simulink model "LATC_Test_Calc"  (R2021b)
settings: Solver=FixedStepDiscrete  StartTime=0.0  StopTime=inf  FixedStep=0.01  RelTol=1e-3
undefined symbols (not defined in the file or in its folder): P_LCS_A0_Dis_BP, P_LCS_A2_Curve_BP, P_LCS_A2S_FliterTime, P_LCS_DeltaEps_SpdBp, P_LCS_LCC_A0_Dis_BP, P_LCS_LCC_AngleSlope_ELK, P_LCS_LCC_AngleSlope_ESS, P_LCS_LCC_AngleSlope_LCCancle, P_LCS_LCC_AngleSlope_LCEco, P_LCS_LCC_AngleSlope_LCK, P_LCS_LCC_AngleSlope_LCKIE, P_LCS_LCC_AngleSlope_LCNomal, P_LCS_LCC_AngleSlope_LCSport, P_LCS_LCC_AngleSlope_LKA, P_LCS_LCC_Eco_AyDtLimit_TBL, P_LCS_LCC_ELK_AyDtLimit_TBL, P_LCS_LCC_ESS_AyDtLimit_TBL, P_LCS_LCC_LC_AyDtLimit_TBL, P_LCS_LCC_LC_Normal_AyDtLimit_TBL, P_LCS_LCC_LC_Planning_Dist_TBL, P_LCS_LCC_LCK_AyDtLimit_TBL, P_LCS_LCC_LCK_Planning_Dist_TBL, P_LCS_LCC_LKA_AyDtLimit_TBL, P_LCS_LCC_Matrix_q1_st, P_LCS_LCC_Matrix_q2_st, P_LCS_LCC_Max_Lateral_Acc_ms2, P_LCS_LCC_MaxLatAcc_ELK, P_LCS_LCC_MaxLatAcc_ESS, P_LCS_LCC_MaxLatAcc_LCCancel, P_LCS_LCC_MaxLatAcc_LCEco, P_LCS_LCC_MaxLatAcc_LCK, P_LCS_LCC_MaxLatAcc_LCKIE, P_LCS_LCC_MaxLatAcc_LCNomal, P_LCS_LCC_MaxLatAcc_LCSport, P_LCS_LCC_MaxLatAcc_LKA, P_LCS_LCC_Min_Plan_Dis, P_LCS_LCC_PlaningLength_m, P_LCS_LCC_PreCur_Min_Plan_Dis_Fac, P_LCS_LCC_PreView_Fac, P_LCS_LCC_PreView_s, P_LCS_LCC_PreViewCurve_Fac, P_LCS_LCC_PreViewT, P_LCS_LCC_Spd_BP, P_LCS_LCC_Spd_BP2, P_LCS_LCC_Sport_AyDtLimit_TBL, P_LCS_LCC_StateActiv_AyDtLimit, P_LCS_LCC_StateActiv_PreviewT, P_LCS_LCC_StateActiveDelaytime, P_LCS_LCC_TarSteerAngleSlope, P_LCS_preDis_spd, P_LCS_StateActiv_AngleSlope, P_LCS_StateActive_HoldTime_BP, P_LCS_StateActiveFlg_BP, P_LCS_StateHold_time
libraries: canapelib x35, simulink x2
(part 3 of 3)

== matlab function LATC_Test_Calc/MATLAB Function1 ==
  data: LineValid input; SteerAngle input; steer_angle output size=[1,1]; Veh_Speed input; ref_curvature input; lateral_error input; lateral_error_rate input; heading_error input; heading_error_rate input; steer_feedforward_temp output; steer_feedbackward_temp output; Left_steer_ratio input; Right_steer_ratio input; Matrix_q1 input; Matrix_q3 input; Max_lateral_acceleration input; TarSteerAngleSlope input; CurrentSteerAngleOffset input; steer_limit_temp output; steer_angleK1 input
function [steer_angle,steer_feedforward_temp,steer_feedbackward_temp,steer_limit_temp]= LQR_Algorithm(LineValid,SteerAngle,Veh_Speed,ref_curvature,lateral_error,lateral_error_rate,heading_error,heading_error_rate,...
    Left_steer_ratio,Right_steer_ratio,Matrix_q1,Matrix_q3,Max_lateral_acceleration,TarSteerAngleSlope,CurrentSteerAngleOffset,steer_angleK1)
if LineValid
    %% 1.车辆参数
    %1.1 车的大小及长度参数
    veh_params.vehicle_length = single(4.875);
    veh_params.vehicle_width  = single(2.2);
    veh_params.vehicle_height = single(1.69);
    %1.2 车辆控制参数
    veh_params.wheel_base = single(2.92);               %轴距, m
    veh_params.Vch = 23.5;                              %特征车速
    veh_params.max_steer_angle = single(53 / 180 * pi); %前轮最大转角
    veh_params.max_acceleration = single(2);            %车辆最大加速度
    veh_params.max_deceleration = single(-2);           %车辆最大减速度
    veh_params.left_steer_ratio = Left_steer_ratio;     %车辆左侧转向传动比%
    veh_params.right_steer_ratio = Right_steer_ratio;   %车辆右侧转向传动比%
    veh_params.cf = single(155494.663);                 %车辆前轮侧偏刚度
    veh_params.cr = single(155494.663);                 %车辆后轮侧偏刚度 
    veh_params.mass_fl = single(520);                   %车辆左前轮负重
    veh_params.mass_fr = single(520);                   %车辆右前轮负重
    veh_params.mass_rl = single(520);                   %车辆左后轮负重
    veh_params.mass_rr = single(520);                   %车辆右后轮负重
    %% 2.控制参数计算
    mass_front =  veh_params.mass_fl + veh_params.mass_fr;
    mass_rear  =  veh_params.mass_rl + veh_params.mass_rr;
    mass =  mass_front + mass_rear;
    lf = veh_params.wheel_base * (single(1.0) - mass_front / mass);
    lr = veh_params.wheel_base * (single(1.0) - mass_rear / mass);
    iz = lf * lf * mass_front + lr * lr * mass_rear;
    %% 3.LQR参数设置
    
    lqr_eps = single(0.01);
    lqr_max_iteration = single(800);
    
    basic_state_size = uint8(4);
    control_size = uint8(1);
    
    matrix_a=  single(zeros(basic_state_size,basic_state_size));
    matrix_a_coeff = single(zeros(basic_state_size,basic_state_size));
    I = single(eye(basic_state_size,basic_state_size));
    matrix_a(1,2) = single(1.0);
    matrix_a(2,3) = single((veh_params.cf + veh_params.cr ) / mass);
    matrix_a(3,4) = single(1.0);
    matrix_a(4,3) = single((lf * veh_params.cf - lr * veh_params.cr) / iz);
    
    matrix_a_coeff(2,2) = single(-(veh_params.cf + veh_params.cr) / mass);
    matrix_a_coeff(2,4) = single(-1.0 * (lr * veh_params.cr + lf * veh_params.cf) / mass);
    matrix_a_coeff(3,4) = single(1.0);
    matrix_a_coeff(4,2) = single((lr * veh_params.cr - lf * veh_params.cf) / iz);
    matrix_a_coeff(4,4) = single(-1.0 * (lf * lf * veh_params.cf + lr * lr * veh_params.cr)/iz);
    
    matrix_a(2,2) = matrix_a_coeff(2,2);
    matrix_a(2,4) = matrix_a_coeff(2,4);
    matrix_a(4,2) = matrix_a_coeff(4,2);
    matrix_a(4,4) = matrix_a_coeff(4,4);
    
    matrix_b = single(zeros(basic_state_size,control_size));
    matrix_b(2,1) = veh_params.cf/mass;
    matrix_b(4,1) = lf * veh_params.cf /iz;
    
    matrix_q = single(zeros(4,4));
    matrix_q(1,1) = Matrix_q1;                      %调整q矩阵的第一、三个参数，改善转向性能0.0001,0.02
    matrix_q(3,3) = Matrix_q3;
    
    lqr_params.A = matrix_a;
    lqr_params.B = matrix_b;
    lqr_params.I = I;
    lqr_params.ts = single(0.02);
    lqr_params.lr = lr;
    lqr_params.lf = lf;
    lqr_params.cf=veh_params.cf;
    lqr_params.cr=veh_params.cf;
    lqr_params.iz=iz;
    lqr_params.mass=mass;
    lqr_params.Q =matrix_q ;
    lqr_params.R = eye(1,1);
    lqr_params.eps=lqr_eps;
    lqr_params.max_iteration=lqr_max_iteration;
    %% 4.计算前轮转角
    lqr_params.A(2,2) = lqr_params.A(2,2)/(max(Veh_Speed, single(0.2)));
    lqr_params.A(2,4) = lqr_params.A(2,4)/(max(Veh_Speed, single(0.2)));
    lqr_params.A(4,2) = lqr_params.A(4,2)/(max(Veh_Speed, single(0.2)));
    lqr_params.A(4,4) = lqr_params.A(4,4)/(max(Veh_Speed, single(0.2)));
    
    A=lqr_params.A;
    B=lqr_params.B;
    I=lqr_params.I;
    ts=lqr_params.ts;
    min_tol = lqr_params.eps;
    max_iter = lqr_params.max_iteration;
    matrix_Q = lqr_params.Q;
    matrix_R = lqr_params.R;
    
    matrix_ad=single(zeros(size(A)));
    matrix_ad=(I+ts*single(0.5) * A) / (I-ts*single(0.5) * A);
    
    matrix_bd=single(zeros(size(B)));
    matrix_bd=B*ts;
    matrix_k = SolveLQRProblem(matrix_ad, matrix_bd, matrix_Q,matrix_R, min_tol, max_iter);
    
    matrix_state = single(zeros(4, 1));
    matrix_state(1, 1) = lateral_error;
    matrix_state(2, 1) = lateral_error_rate;
    matrix_state(3, 1) = heading_error;
    matrix_state(4, 1) = heading_error_rate;
    steer_feedbackward = -(matrix_k * matrix_state);
    % 前馈转角
    kv = lqr_params.lr * lqr_params.mass / single(1) / lqr_params.cf / veh_params.wheel_base - ...
        lqr_params.lf * lqr_params.mass / single(1) / lqr_params.cr / veh_params.wheel_base;
    steer_feedforward = (veh_params.wheel_base * ref_curvature + kv * Veh_Speed * Veh_Speed * ref_curvature - matrix_k(1, 3) * ...
        (lqr_params.lr * ref_curvature - lqr_params.lf * lqr_params.mass * Veh_Speed * Veh_Speed * ref_curvature / single(1) / lqr_params.cr / veh_params.wheel_base));%弧度制角度rad
    % 4.3 计算期望前轮偏角
    steer_cmd = steer_feedforward + steer_feedbackward;
    
    if (steer_cmd>=0)
        steer_transmission_ratio = veh_params.left_steer_ratio;
    else
        steer_transmission_ratio = veh_params.right_steer_ratio;
    end
    steer_feedforward_temp = steer_feedforward * single(57.3) * steer_transmission_ratio;%反算方向盘转角并转换为角度制deg
    steer_feedbackward_temp = steer_feedbackward * single(57.3) * steer_transmission_ratio;%反算方向盘转角并转换为角度制deg
    steer_angle_cmd = steer_cmd * single(57.3) * steer_transmission_ratio;%反算方向盘转角并转换为角度制deg
    %% 5.限制期望前轮偏角
    % 5.1 根据横向加速度限制前轮转角
    if Veh_Speed < 1
        steer_limit = atan( Max_lateral_acceleration * veh_params.wheel_base /(Veh_Speed *Veh_Speed))* single(57.3) * steer_transmission_ratio; % 高速计算不准确，更改为下面特征车速计算方法
    else
        AckConst = min((single(1)+Veh_Speed*Veh_Speed/(veh_params.Vch*veh_params.Vch))*veh_params.wheel_base/max(single(1),Veh_Speed),single(32767));
        % PsiDtAckRaw = (SteerAngle/steer_transmission_ratio)/AckConst;
        steer_limit = ((Max_lateral_acceleration * AckConst)/Veh_Speed)* single(57.3) * steer_transmission_ratio;
    end
    %     steer_limit = atan( Max_lateral_acceleration * veh_params.wheel_base /(Veh_Speed *Veh_Speed)) * steer_transmission_ratio;
    steer_angle_cmd = min(steer_limit, max(-steer_limit,steer_angle_cmd));%方向盘角度制deg
    
    steer_angle_deg = steer_angle_cmd;
    steer_limit_temp = steer_limit;
    % 5.2 限制方向盘转速
    steer_angle = min(steer_angleK1 + TarSteerAngleSlope,max(steer_angleK1 - TarSteerAngleSlope,steer_angle_deg));
    
else
    steer_angle = SteerAngle-CurrentSteerAngleOffset;
    steer_feedforward_temp = single(0);
    steer_feedbackward_temp = single(0);
    steer_limit_temp = single(0);
end
end

== matlab function LATC_Test_Calc/Motion_Planning/FrenetTrajectory_Lateral/Subsystem/MATLAB Function ==
  data: Forward_PreViewT input; VehSpd input; PreCurve output; C2 input; C3 input
function PreCurve = PreView_Point_Curvature(Forward_PreViewT,VehSpd,C2,C3)
LookForwardDis = VehSpd * Forward_PreViewT;
PreCurve = 6*C3*LookForwardDis + 2*C2;
end

== matlab function LATC_Test_Calc/Motion_Planning/FrenetTrajectory_Lateral/Subsystem/MATLAB Function1 ==
  data: Delaytime input uint16; Flg output uint8; Count output uint16; TarDangerLevel input uint8; TarDangerLevelK1 input uint8; FlgK1 input uint8; CountK1 input uint16
function [Flg,Count]= fcn(Delaytime,TarDangerLevel,TarDangerLevelK1,FlgK1,CountK1)
Count = min(CountK1 + uint16(1),Delaytime);
if Count == Delaytime
    Flg = uint8(0);
else
    Flg = FlgK1;
end
%%状态检测
if TarDangerLevel == uint8(1) && TarDangerLevelK1 == 0 %功能激活
    Count = uint16(0);
    Flg = uint8(1);  
end
end

== matlab function LATC_Test_Calc/Motion_Planning/CartesianTrajectory/FrenetTrajectory ==
  data: A0 input; A1 input; A2 input; A3 input; Veh_Speed input size=1; YawRate input size=1; TarDangerlLevel input; PreView_T input size=1; PlanX output; PlanY output; PlanTheta output; idx output; PreviewX output; PreviewY output; PreviewTheta output; numTraj output size=1; ref_curvature output; AyDtLimit input size=1; Min_Plan_Dis input; lateral_error output size=1; lateral_error_rate output size=1; heading_error output size=1; heading_error_rate output size=1; axEgo input; kapEgo input
function [PlanX,PlanY,PlanTheta,idx,PreviewX,PreviewY,PreviewTheta,numTraj,ref_curvature,lateral_error,lateral_error_rate,heading_error,heading_error_rate] ...
    = FrenetTrajectory(A0,A1,A2,A3,Veh_Speed,YawRate,TarDangerlLevel,PreView_T,AyDtLimit,Min_Plan_Dis,axEgo,kapEgo)
%% 生成轨迹
Px =single([1.5 2 2.5 2.7 3 3.3 3.6 4 4.4 4.8 5.3 5.8 6.4 7.1 7.8 8.6 9.5 10.4 11.4]); %Py_Fac后期去掉，增加一个轨迹筛选条件，每个车速下最小规划距离
TarEgoAx = zeros(1,length(Px));
TarEgoV = ones(1,length(Px)) .* Veh_Speed;
if Veh_Speed>single(1)
    Px = Veh_Speed*Px;
end
Py = A3*(Px.^3) + A2*(Px.^2) + A1*(Px.^1) + A0;
x = single(zeros(11,1));
y = single(zeros(11,1));
Vx = single(zeros(11,1));
Vy = single(zeros(11,1));
Ax = single(zeros(11,1));
Ay = single(zeros(11,1));
AyDt = single(zeros(11,1));
Pt = single(zeros(1,1));
for i = 1:length(Py)
    Pt = 1.05*sqrt(Px(i)^2 + Py(i)^2)/max(1,0.5*(TarEgoV(i) + Veh_Speed));
    t_Vego = max(Veh_Speed,1);
    t0 = single(0);
    tn = Pt;
    T = [t0^5,t0^4,t0^3,t0^2,t0,1;...
        5*t0^4,4*t0^3,3*t0^2,2*t0,1,0;...
        20*t0^3,12*t0^2,6*t0,2,0,0;...
        tn^5,tn^4,tn^3,tn^2,tn,1;...
        5*tn^4,4*tn^3,3*tn^2,2*tn,1,0;...
        20*tn^3,12*tn^2,6*tn,2,0,0];
    Vn = TarEgoV(i);
    An = TarEgoAx(i);
    kP =  3*A3*(Px(i).^2) + 2*A2*Px(i) + A1;
    
    Kap = 6*A3*(Px(i))+2*A2;
    Arcf = (Veh_Speed^2)*Kap;
    Ayn = Arcf/sqrt(1 + kP^2);
    Axn = Arcf*kP/sqrt(1 + kP^2);
    
    Vxn = Vn/sqrt(1 + kP^2);
    Vyn = Vn*kP/sqrt(1 + kP^2);
    MaX = [0;t_Vego;axEgo;Px(i);Vxn;Axn];
    MaY = [0;0;(Veh_Speed^2)*kapEgo;Py(i);Vyn;Ayn];
    A = T\MaX;
    B = T\MaY;
    
    a5 = A(1); % 纵向轨迹系数
    a4 = A(2);
    a3 = A(3);
    a2 = A(4);
    a1 = A(5);
    a0 = A(6);
    
    b5 = B(1); % 横向轨迹系数
    b4 = B(2);
    b3 = B(3);
    b2 = B(4);
    b1 = B(5);
    b0 = B(6);
    preLineValid = true;
    for j=1:11
        t = (j-1)*tn/10;
        x(j) = a5*t^5 + a4*t^4 + a3*t^3 + a2*t^2 + a1*t + a0;
        Vx(j) = 5*a5*t^4 + 4*a4*t^3 + 3*a3*t^2 + 2*a2*t + a1;
        Ax(j) = 20*a5*t^3 + 12*a4*t^2 + 6*a3*t + 2*a2;
        y(j) = b5*t^5 + b4*t^4 + b3*t^3 + b2*t^2 + b1*t + b0;
        Vy(j) = 5*b5*t^4 + 4*b4*t^3 + 3*b3*t^2 + 2*b2*t + b1;
        Ay(j) = 20*b5*t^3 + 12*b4*t^2 + 6*b3*t + 2*b2;
        AyDt(j) = 60*b5*t^2 + 24*b4*t + 6*b3;
        if abs(AyDt(j))>AyDtLimit 
            preLineValid = false;
            break;
        end     
    end
    if abs(sqrt(x(11)^2+y(11)^2)) < Min_Plan_Dis
       preLineValid = false; 
    end
    if preLineValid
        break;
    end
end
NumTarpoints = 40;
y = y.*single(-1);
objSpline = Spline2D(y,x);
s = single(linspace(0,objSpline.s(end),NumTarpoints));
TargetPoints = single(zeros(length(s),6));
for i = single(1):single(1):length(s)
    [ix,iy] = objSpline.calc_position(s(i));
    TargetPoints(i,1) = ix;
    TargetPoints(i,2) = iy;
    TargetPoints(i,3) = objSpline.calc_yaw(s(i));
    TargetPoints(i,4) = objSpline.calc_curvature(s(i));
    TargetPoints(i,5) = objSpline.calc_curvatureDerivative(s(i));
    TargetPoints(i,6) = s(i);
end
traj = single(zeros(NumTarpoints,6)); t= single(zeros(NumTarpoints,1)); costs = single(zeros(1,1));
globalTrajectory = repmat(struct('Trajectory',traj,'Times',t,'costs',costs), 1, 1);
globalTrajectory(1).Trajectory = TargetPoints;
globalTrajectory(1).Times = t;

numTraj  = i;%借用numTraj输出时间点索引号
%%
% [s,d]→[x, y, theta, kappa, dkappa]
PlanX= globalTrajectory(1).Trajectory(1:NumTarpoints,2);
PlanY= globalTrajectory(1).Trajectory(1:NumTarpoints,1);
PlanTheta = globalTrajectory(1).Trajectory(1:NumTarpoints,3);
[matrix_state,ref_curvature,idx] = Calc_State_Error(Veh_Speed,YawRate,globalTrajectory,PreView_T,NumTarpoints);
PreviewX = globalTrajectory(1).Trajectory(idx,2);
PreviewY = globalTrajectory(1).Trajectory(idx,1);
PreviewTheta = globalTrajectory(1).Trajectory(idx,3);
% lateral_error = single(zeros(1,1));lateral_error_rate = single(zeros(1,1));heading_error = single(zeros(1,1));heading_error_rate = single(zeros(1,1));
lateral_error = matrix_state(1,1);
lateral_error_rate = matrix_state(2,1);
heading_error = matrix_state(3,1);
heading_error_rate = matrix_state(4,1);

end

== matlab function LATC_Test_Calc/Motion_Planning/CartesianTrajectory/Subsystem/MATLAB Function ==
  data: Forward_PreViewT input; VehSpd input; PreCurve output; C2 input; C3 input
function PreCurve = PreView_Point_Curvature(Forward_PreViewT,VehSpd,C2,C3)
LookForwardDis = VehSpd * Forward_PreViewT;
PreCurve = 6*C3*LookForwardDis + 2*C2;
end

== matlab function LATC_Test_Calc/Motion_Planning/CartesianTrajectory/Subsystem/MATLAB Function1 ==
  data: Delaytime input uint16; Flg output uint8; Count output uint16; TarDangerLevel input uint8; TarDangerLevelK1 input uint8; FlgK1 input uint8; CountK1 input uint16
function [Flg,Count]= fcn(Delaytime,TarDangerLevel,TarDangerLevelK1,FlgK1,CountK1)
Count = min(CountK1 + uint16(1),Delaytime);
if Count == Delaytime
    Flg = uint8(0);
else
    Flg = FlgK1;
end
%%状态检测
if TarDangerLevel == uint8(1) && TarDangerLevelK1 == 0 %功能激活
    Count = uint16(0);
    Flg = uint8(1);  
end
end

== matlab function LATC_Test_Calc/Motion_Planning/FrenetTrajectory_Lateral/Subsystem1/MATLAB Function ==
  data: Forward_PreViewT input; VehSpd input; PreCurve output; C2 input; C3 input
function PreCurve = PreView_Point_Curvature(Forward_PreViewT,VehSpd,C2,C3)
LookForwardDis = VehSpd * Forward_PreViewT;
PreCurve = 6*C3*LookForwardDis + 2*C2;
end

== matlab function LATC_Test_Calc/Motion_Planning/FrenetTrajectory_Lateral/Subsystem1/MATLAB Function1 ==
  data: Delaytime input uint16; Flg output uint8; Count output uint16; TarDangerLevel input uint8; TarDangerLevelK1 input uint8; FlgK1 input uint8; CountK1 input uint16
function [Flg,Count]= fcn(Delaytime,TarDangerLevel,TarDangerLevelK1,FlgK1,CountK1)
Count = min(CountK1 + uint16(1),Delaytime);
if Count == Delaytime
    Flg = uint8(0);
else
    Flg = FlgK1;
end
%%状态检测
if TarDangerLevel == uint8(1) && TarDangerLevelK1 == 0 %功能激活
    Count = uint16(0);
    Flg = uint8(1);  
end
end

== matlab function LATC_Test_Calc/SteerAngSlopeCalc/MATLAB Function3 ==
  data: delytime input uint16; TarDangerLevel input uint8; TarDangerLevelK1 input uint8; FLg output uint8; FLgK1 input uint8; CntK1 input uint16; Cnt output uint16
function [FLg,Cnt] = AngSlopeCalc(delytime,TarDangerLevel,TarDangerLevelK1,FLgK1,CntK1)

Cnt = min(CntK1 + uint16(1),delytime);
if Cnt== delytime
    FLg = uint8(0);
else
    FLg = FLgK1;
end
%FLg = FLgK1;
%% 
if TarDangerLevel==uint8(1) && TarDangerLevelK1==0  % NO function 2 LCK (TarDangerLevelK1==0)
    Cnt =uint16(0);
    FLg = uint8(1);
end

if  TarDangerLevel==uint8(3) && (TarDangerLevelK1==uint8(1)||TarDangerLevelK1==uint8(2)) % LCK/IE 2 LC_Normal
    Cnt =uint16(0);
    FLg = uint8(2);
end

if  TarDangerLevel==uint8(7) && (TarDangerLevelK1==uint8(1)||TarDangerLevelK1==uint8(2)) % LCK/IE 2 LC_Eco
    Cnt =uint16(0);
    FLg = uint8(3);
end

if  TarDangerLevel==uint8(8) && (TarDangerLevelK1==uint8(1)||TarDangerLevelK1==uint8(2)) % LCK/IE 2 LC_sport
    Cnt =uint16(0);
    FLg = uint8(4);
end
if  TarDangerLevel==uint8(6) && (TarDangerLevelK1==uint8(1)||TarDangerLevelK1==uint8(2)) % LCK/IE 2 ESS 后期添加配和ESS Slope 一起调试
    Cnt =uint16(0);
    FLg = uint8(5);
end

== matlab function LATC_Test_Calc/Motion_Planning/FrenetTrajectory_Lateral/FrenetTrajectory_Lateral ==
  data: A0 input; A1 input; A2 input; A3 input; Veh_Speed input size=1; YawRate input size=1; TarDangerlLevel input; PreView_T input size=1; PlanX output; PlanY output; PlanTheta output; idx output; PreviewX output; PreviewY output; PreviewTheta output; numTraj output size=1; ref_curvature output; AyDtLimit input size=1; Min_Plan_Dis input; lateral_error output size=1; lateral_error_rate output size=1; heading_error output size=1; heading_error_rate output size=1
function [PlanX,PlanY,PlanTheta,idx,PreviewX,PreviewY,PreviewTheta,numTraj,ref_curvature,lateral_error,lateral_error_rate,heading_error,heading_error_rate] ...
    = FrenetTrajectory_Lateral(A0,A1,A2,A3,Veh_Speed,YawRate,TarDangerlLevel,PreView_T,AyDtLimit,Min_Plan_Dis)
Veh_Speed = max(Veh_Speed,2);
%% 参考线离散化
rx1 = [single(0):single(1):single(19)];
rx2 = [single(20):20:150];
rx = cat(2,rx1,rx2);
ry = single((-1)).*(A0 + A1.* rx + A2.* (rx.^2) + A3.* (rx.^3));
waypoints = [ry',rx'];
referencePathPointNum = 100;
referencePath = FrenentReferencePath(waypoints,referencePathPointNum);
pathStart = referencePath.interpolate(0);% 求起始点处车辆状态 [x, y,theta, kappa, dkappa, s]
initialState=[0 -A0 pathStart(1,3)];

Frenet_traj_obj = TrajectoryGeneratorFrenet(referencePath);
FtNumTarpoints = single(40); % Frenet坐标系轨迹点数
GtNumTarpoints = single(40); % 全局坐标系轨迹点数
%% 生成轨迹
Py =single([1.5 2 2.5 3 3.6 4.4 5 5.8 6.4 7	7.8	8.6	9.5 10.4 11.4]);% 按等比1.1
Py = max(Veh_Speed,5) .* Py; % 暂时设定最短规划距离 5*2.5
Px = single((-1)).*(A3.*(Py.^3) + A2.*(Py.^2) + A1.*(Py.^1) + A0);
for i = 1:length(Py)
    arcLenOffsets = 1.05*sqrt(Px(i)^2 + Py(i)^2);
    [frenetTrajectory,globalTrajectory,numTraj] = Frenet_traj_obj.FrenetTrajectory_Lateral(initialState,arcLenOffsets,0,FtNumTarpoints,GtNumTarpoints);
    AyDt = (diff(frenetTrajectory.Trajectory(:,3).*(Veh_Speed*Veh_Speed)))./diff(frenetTrajectory.Trajectory(:,1)./Veh_Speed);
    if all(abs(AyDt(1:end,1)) < AyDtLimit) && (frenetTrajectory.Trajectory(end,1) > Min_Plan_Dis)
        break;
    end
end
numTraj = i;%借用numTraj将第几个时间点输出
[globalTrajectory] = EvaluateTrajectory_Lateral(frenetTrajectory,globalTrajectory, 1,1);
%%
% [s,d]→[x, y, theta, kappa, dkappa]
PlanX = single(zeros(GtNumTarpoints,1));
PlanY = single(zeros(GtNumTarpoints,1));
PlanTheta = single(zeros(GtNumTarpoints,1));
PlanX= globalTrajectory(1).Trajectory(1:GtNumTarpoints,2);
PlanY= globalTrajectory(1).Trajectory(1:GtNumTarpoints,1);
PlanTheta = globalTrajectory(1).Trajectory(1:GtNumTarpoints,3);
[matrix_state,ref_curvature,idx] = Calc_State_Error(Veh_Speed,YawRate,globalTrajectory,PreView_T,GtNumTarpoints);
PreviewX = globalTrajectory(1).Trajectory(idx,2);
PreviewY = globalTrajectory(1).Trajectory(idx,1);
PreviewTheta = globalTrajectory(1).Trajectory(idx,3);
% lateral_error = single(zeros(1,1));lateral_error_rate = single(zeros(1,1));heading_error = single(zeros(1,1));heading_error_rate = single(zeros(1,1));
lateral_error = matrix_state(1,1);
lateral_error_rate = matrix_state(2,1);
heading_error = matrix_state(3,1);
heading_error_rate = matrix_state(4,1);

end

== matlab function LATC_Test_Calc/Motion_Planning/FrenetTrajectory_Lateral_CalcA0/Subsystem/MATLAB Function ==
  data: Forward_PreViewT input; VehSpd input; PreCurve output; C2 input; C3 input
function PreCurve = PreView_Point_Curvature(Forward_PreViewT,VehSpd,C2,C3)
LookForwardDis = VehSpd * Forward_PreViewT;
PreCurve = 6*C3*LookForwardDis + 2*C2;
end

== matlab function LATC_Test_Calc/Motion_Planning/FrenetTrajectory/FrenetTrajectory ==
  data: A0 input; A1 input; A2 input; A3 input; Veh_Speed input size=1; YawRate input size=1; TarDangerlLevel input; PreView_T input size=1; PlanX output; PlanY output; PlanTheta output; idx output; PreviewX output; PreviewY output; PreviewTheta output; numTraj output size=1; ref_curvature output; AyDtLimit input size=1; Min_Plan_Dis input; lateral_error output size=1; lateral_error_rate output size=1; heading_error output size=1; heading_error_rate output size=1
function [PlanX,PlanY,PlanTheta,idx,PreviewX,PreviewY,PreviewTheta,numTraj,ref_curvature,lateral_error,lateral_error_rate,heading_error,heading_error_rate] ...
    = FrenetTrajectory(A0,A1,A2,A3,Veh_Speed,YawRate,TarDangerlLevel,PreView_T,AyDtLimit,Min_Plan_Dis)
% 参考线离散化
rx1 = [single(0):single(1):single(19)];
rx2 = [single(20):20:150];
rx = cat(2,rx1,rx2);
ry = single((-1)).*(A0 + A1.* rx + A2.* (rx.^2) + A3.* (rx.^3));
waypoints = [ry',rx'];
referencePathPointNum = 100; %参考轨迹的点的个数(参考点的分辨率)，此参数会影响最终目标轨迹线的形状，太小会出现轨迹线拐点
referencePath = FrenentReferencePath(waypoints,referencePathPointNum);
% pathStart = referencePath.interpolate(0);% 求起始点处车辆状态 [x, y,theta, kappa, dkappa, s],车辆在起始点处。%删除此种办法，经过测试发现在弯道或者换道过程中，A1项大的时候轨迹存往反方向突出一点再返回的问题
%% 定义轨迹起始点状态
initGlobalState = [0 0 pi/2 0 Veh_Speed  0]; %暂时定义纵向加速度为0，[x, y,theta, kappa speed，Acc]
initFrenetState = referencePath.global2frenet(initGlobalState);
% Py =single([2.5	2.7	3 3.3 3.6 4 4.4	4.8	5.3	5.8	6.4	7.1	7.8	8.6	9.5 10.4 11.4].*Py_Fac);
Py =single([1.5 2 2.5 3 3.6 4.2 5 5.8 6.4 7	7.8	8.6	9.5 10.4 11.4]);
TarEgoAy = zeros(1,length(Py));% 终点处期望纵向加速度
TarEgoV = ones(1,length(Py)) .* Veh_Speed;% 终点处期望纵向速度
Py = max(Veh_Speed,5).*Py;
Px = single((-1)).*(A3.*(Py.^3) + A2.*(Py.^2) + A1.*(Py.^1) + A0);

Frenet_traj_obj = TrajectoryGeneratorFrenet(referencePath);
FtNumTarpoints = single(40); % Frenet坐标系轨迹点数
%% 生成轨迹
for i = 1:length(Py)
    Pl = round(1.05*sqrt(Px(i)^2 + Py(i)^2));
    Pt = round(1.05*sqrt(Px(i)^2 + Py(i)^2)/max(1,0.5*(TarEgoV(i) + Veh_Speed)));
    pathend= referencePath.interpolate(Pl);
    EndGlobalState = [pathend(1:4) TarEgoV(i) TarEgoAy(i)];
    EndFrenetState = referencePath.global2frenet(EndGlobalState);
    [frenetTrajectory,globalTrajectory] = Frenet_traj_obj.FrenetTrajectory(initFrenetState,EndFrenetState(1,1),0,EndFrenetState(1,2:3),EndFrenetState(1,5:6),Pt,FtNumTarpoints);
    AyDt = abs(diff(globalTrajectory.Trajectory(:,4).*((globalTrajectory.Trajectory(:,5).^2)))./diff(globalTrajectory.Times));
    if all(abs(AyDt)<AyDtLimit) && (frenetTrajectory.Trajectory(end,1) > Min_Plan_Dis)
        break;
    end
end
numTraj  = i;%借用numTraj输出时间点索引号
[globalTrajectory] = EvaluateTrajectory(frenetTrajectory,globalTrajectory,1,1,1,1);
%%
% [s,d]→[x, y, theta, kappa, dkappa]
PlanX = single(zeros(FtNumTarpoints,1));
PlanY = single(zeros(FtNumTarpoints,1));
PlanTheta = single(zeros(FtNumTarpoints,1));
PlanX= globalTrajectory(1).Trajectory(1:FtNumTarpoints,2);
PlanY= globalTrajectory(1).Trajectory(1:FtNumTarpoints,1);
PlanTheta = globalTrajectory(1).Trajectory(1:FtNumTarpoints,3);
[matrix_state,ref_curvature,idx] = Calc_State_Error(Veh_Speed,YawRate,globalTrajectory,PreView_T,FtNumTarpoints);
PreviewX = globalTrajectory(1).Trajectory(idx,2);
PreviewY = globalTrajectory(1).Trajectory(idx,1);
PreviewTheta = globalTrajectory(1).Trajectory(idx,3);
% lateral_error = single(zeros(1,1));lateral_error_rate = single(zeros(1,1));heading_error = single(zeros(1,1));heading_error_rate = single(zeros(1,1));
lateral_error = matrix_state(1,1);
lateral_error_rate = matrix_state(2,1);
heading_error = matrix_state(3,1);
heading_error_rate = matrix_state(4,1);

end
